simulink model "rtds"  (R2015a)
settings: Solver=ode45  StartTime=0.0  StopTime=100.0  RelTol=1e-3
undefined symbols (not defined in the file): AXI4, Lite
libraries: xbsIndex_r4 x73, s2ss x1
Description:
  | This is my first test model!
settings Model: Creator=ACS  LastModifiedBy=ACS

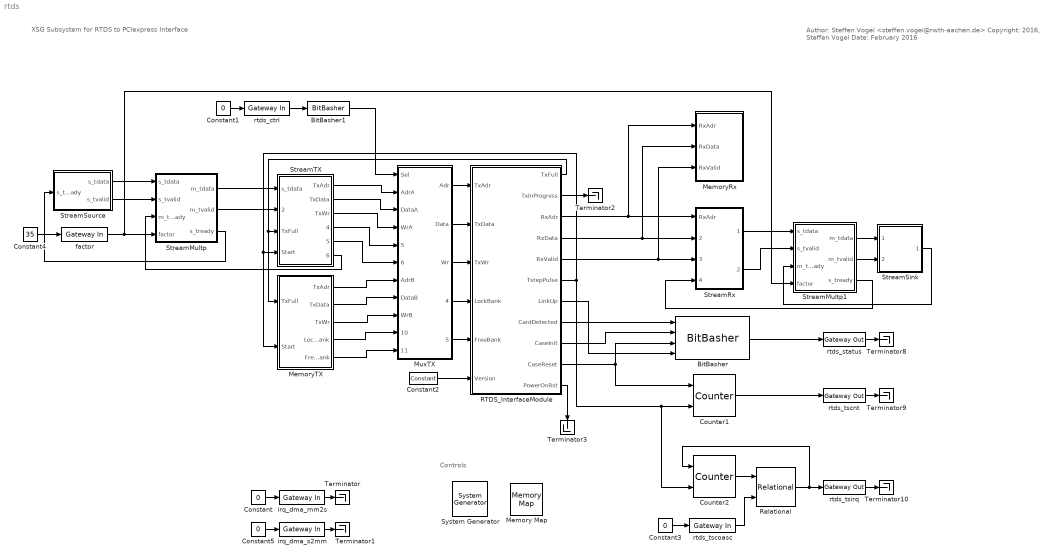
== system rtds ==
  note: XSG Subsystem for RTDS to PCIexpress Interface
  note: Author: Steffen Vogel <steffen.vogel@rwth-aachen.de>
      | Copyright: 2016, Steffen Vogel
      | Date: February 2016
  note: Controls
  " System Generator" : xbsIndex_r4/ System Generator  Tag=genX  xilinxfamily=virtex7  part=xc7vx485t  speed=-2  package=ffg1761  synthesis_tool=Vivado  clock_wrapper=Clock Enables  directory=D:/msv/02_msv-svo/s2ss/clients/sysgen/example/compiled/rtds2  proj_type=Vivado  Synth_file=Vivado Synthesis Defaults  Impl_file=Vivado Implementation Defaults  testbench=off  simulink_period=1  sysclk_period=8  dcm_input_clock_period=10  incr_netlist=off  trim_vbits=Everywhere in SubSystem  dbl_ovrd=According to Block Masks  core_generation=According to Block Masks  run_coregen=off  deprecated_control=off  eval_field=0  block_type=sysgen
  BitBasher : xbsIndex_r4/BitBasher  bitexpr=status={link_up,card_detected,case_reset,case_init}  display_expr=off  sr_1=status  arith_type1=Unsigned  bin_pt1=0  sr_2=2  arith_type2=Unsigned  bin_pt2=0  sr_3=3  arith_type3=Unsigned  bin_pt3=0  sr_4=4  arith_type4=Unsigned  bin_pt4=0  dbl_ovrd=off  block_type=bitbasher
  BitBasher1 : xbsIndex_r4/BitBasher  bitexpr=sel={ctrl[0]}  display_expr=off  sr_1=sel  arith_type1=Unsigned  bin_pt1=0  sr_2=2  arith_type2=Unsigned  bin_pt2=0  sr_3=3  arith_type3=Unsigned  bin_pt3=0  sr_4=4  arith_type4=Unsigned  bin_pt4=0  dbl_ovrd=off  block_type=bitbasher
  Constant{,1,3,5} (4 alike) : Constant  Value=0
  Constant2 : xbsIndex_r4/Constant  const=3  gui_display_data_type=Fixed-point  arith_type=Signed (2's comp)  n_bits=16  bin_pt=0  preci_type=Single  exp_width=8  frac_width=24  explicit_period=off  period=1  equ=P=C  opselect=C  inp2=PCIN>>17  opr=+  inp1=P  carry=CIN  dbl_ovrd=off  block_type=constant
  Constant4 : Constant  Value=35
  Counter1 : xbsIndex_r4/Counter  cnt_type=Free Running  cnt_to=Inf  operation=Up  start_count=0  cnt_by_val=1  arith_type=Unsigned  n_bits=32  bin_pt=0  load_pin=off  rst=on  en=on  explicit_period=on  period=1  use_behavioral_HDL=off  implementation=Fabric  dbl_ovrd=off  block_type=counter
  Counter2 : xbsIndex_r4/Counter  cnt_type=Free Running  cnt_to=Inf  operation=Up  start_count=0  cnt_by_val=1  arith_type=Unsigned  n_bits=32  bin_pt=0  load_pin=off  rst=on  en=on  explicit_period=on  period=1  use_behavioral_HDL=off  implementation=Fabric  dbl_ovrd=off  block_type=counter
  Memory Map : s2ss/Memory Map  version=1.0  author=Steffen Vogel <stvogel@eonerc.rwth-aachen.de>  desc=System Generator Model  company_url=http://www.acs.eonerc.rwth-aachen.de  vendor=acs.eonerc.rwth-aachen.de  vendor_display_name=Institute for Automation of Complex Power Systems, EONERC, RWTH Aachen University
  MemoryRx : Subsystem
  MemoryTX : Subsystem
  MuxTX : Subsystem
  RTDS_InterfaceModule : Subsystem
  Relational : xbsIndex_r4/Relational  mode=a=b  op_type=Bool  en=off  latency=1  dbl_ovrd=off  block_type=relational
  StreamMultp : Subsystem
  StreamMultp1 : Subsystem
  StreamRx : Subsystem
  StreamSink : Subsystem
  StreamSource : Subsystem
  StreamTX : Subsystem
  Terminator{,1..3,8..10} (7 alike) : Terminator
  factor : xbsIndex_r4/Gateway In  gui_display_data_type=Floating-point  arith_type=Floating-point  n_bits=32  bin_pt=0  preci_type=Single  exp_width=8  frac_width=24  rows=1  columns=1  quantization=Truncate  overflow=Wrap  period=1  UseAsADC=off  ADCChannel='1'  interface=AXI4-Lite  automatic_assignment=on  address_offset=hex2dec('00')  intf_name=''  intf_description=''  timing_constraint=None  locs_specified=off  LOCs={}  io_standard={}  inherit_from_input=off  hdl_port=on  dbl_ovrd=off  block_type=gatewayin
  irq_dma_mm2s : xbsIndex_r4/Gateway In  gui_display_data_type=Boolean  arith_type=Boolean  n_bits=32  bin_pt=0  preci_type=Single  exp_width=8  frac_width=24  rows=1  columns=1  quantization="Round  (unbiased: +/- Inf)"  overflow=Saturate  period=1  UseAsADC=off  ADCChannel='1'  interface=None  automatic_assignment=on  address_offset=hex2dec('00')  intf_name=''  intf_description=''  timing_constraint=None  locs_specified=off  LOCs={}  io_standard={}  inherit_from_input=off  hdl_port=on  dbl_ovrd=off  block_type=gatewayin
  irq_dma_s2mm : xbsIndex_r4/Gateway In  gui_display_data_type=Boolean  arith_type=Boolean  n_bits=32  bin_pt=0  preci_type=Single  exp_width=8  frac_width=24  rows=1  columns=1  quantization="Round  (unbiased: +/- Inf)"  overflow=Saturate  period=1  UseAsADC=off  ADCChannel='1'  interface=None  automatic_assignment=on  address_offset=hex2dec('00')  intf_name=''  intf_description=''  timing_constraint=None  locs_specified=off  LOCs={}  io_standard={}  inherit_from_input=off  hdl_port=on  dbl_ovrd=off  block_type=gatewayin
  rtds_ctrl : xbsIndex_r4/Gateway In  gui_display_data_type=Fixed-point  arith_type=Unsigned  n_bits=32  bin_pt=0  preci_type=Single  exp_width=8  frac_width=24  rows=1  columns=1  quantization="Round  (unbiased: +/- Inf)"  overflow=Saturate  period=1  UseAsADC=off  ADCChannel='1'  interface=AXI4-Lite  automatic_assignment=on  address_offset=hex2dec('00')  intf_name=''  intf_description=''  timing_constraint=None  locs_specified=off  LOCs={}  io_standard={}  inherit_from_input=off  hdl_port=on  dbl_ovrd=off  block_type=gatewayin
  rtds_status : xbsIndex_r4/Gateway Out  inherit_from_input=off  hdl_port=on  rows=1  columns=1  UseAsDAC=off  DACChannel='1'  interface=AXI4-Lite  automatic_assignment=on  address_offset=hex2dec('00')  intf_name=''  intf_description=''  timing_constraint=None  locs_specified=off  LOCs={}  io_standard={}  block_type=gatewayout
  rtds_tscnt : xbsIndex_r4/Gateway Out  inherit_from_input=off  hdl_port=on  rows=1  columns=1  UseAsDAC=off  DACChannel='1'  interface=AXI4-Lite  automatic_assignment=on  address_offset=hex2dec('00')  intf_name=''  intf_description=''  timing_constraint=None  locs_specified=off  LOCs={}  io_standard={}  block_type=gatewayout
  rtds_tscoasc : xbsIndex_r4/Gateway In  gui_display_data_type=Fixed-point  arith_type=Unsigned  n_bits=32  bin_pt=0  preci_type=Single  exp_width=8  frac_width=24  rows=1  columns=1  quantization=Truncate  overflow=Wrap  period=1  UseAsADC=off  ADCChannel='1'  interface=AXI4-Lite  automatic_assignment=on  address_offset=hex2dec('00')  intf_name=''  intf_description=''  timing_constraint=None  locs_specified=off  LOCs={}  io_standard={}  inherit_from_input=off  hdl_port=on  dbl_ovrd=off  block_type=gatewayin
  rtds_tsirq : xbsIndex_r4/Gateway Out  inherit_from_input=off  hdl_port=on  rows=1  columns=1  UseAsDAC=off  DACChannel='1'  interface=Interrupt  automatic_assignment=on  address_offset=hex2dec('00')  intf_name=''  intf_description=''  timing_constraint=None  locs_specified=off  LOCs={}  io_standard={}  block_type=gatewayout
  wires:
  irq_dma_mm2s/1 -> Terminator/1
  RTDS_InterfaceModule/5(RxValid) -> StreamRx/3(RxValid), MemoryRx/3(RxValid)
  BitBasher/1 -> rtds_status/1
  Counter1/1 -> rtds_tscnt/1
  Relational/1 -> Counter2/1, rtds_tsirq/1
  Counter2/1 -> Relational/1
  rtds_tscoasc/1 -> Relational/2
  RTDS_InterfaceModule/10(CaseReset) -> Counter1/1, BitBasher/3
  RTDS_InterfaceModule/4(RxData) -> MemoryRx/2(RxData), StreamRx/2(RxData)
  RTDS_InterfaceModule/8(CardDetected) -> BitBasher/1
  RTDS_InterfaceModule/9(CaseInit) -> BitBasher/2
  RTDS_InterfaceModule/7(LinkUp) -> BitBasher/4
  Constant2/1 -> RTDS_InterfaceModule/6(Version)
  RTDS_InterfaceModule/3(RxAdr) -> MemoryRx/1(RxAdr), StreamRx/1(RxAdr)
  RTDS_InterfaceModule/2(TxInProgress) -> Terminator2/1
  RTDS_InterfaceModule/11(PowerOnRst) -> Terminator3/1
  rtds_status/1 -> Terminator8/1
  rtds_tscnt/1 -> Terminator9/1
  rtds_tsirq/1 -> Terminator10/1
  rtds_ctrl/1 -> BitBasher1/1
  StreamTX/1(TxAdr) -> MuxTX/2(AdrA)
  StreamTX/2(TxData) -> MuxTX/3(DataA)
  StreamTX/3(TxWr) -> MuxTX/4(WrA)
  StreamTX/4(LockBank) -> MuxTX/5(LockBankA)
  StreamTX/5(FreeBank) -> MuxTX/6(FreeBankA)
  BitBasher1/1 -> MuxTX/1(Sel)
  MemoryTX/1(TxAdr) -> MuxTX/7(AdrB)
  MemoryTX/2(TxData) -> MuxTX/8(DataB)
  MemoryTX/3(TxWr) -> MuxTX/9(WrB)
  MemoryTX/4(LockBank) -> MuxTX/10(LockBankB)
  MemoryTX/5(FreeBank) -> MuxTX/11(FreeBankB)
  MuxTX/1(Adr) -> RTDS_InterfaceModule/1(TxAdr)
  MuxTX/2(Data) -> RTDS_InterfaceModule/2(TxData)
  MuxTX/3(Wr) -> RTDS_InterfaceModule/3(TxWr)
  MuxTX/4(LockBank) -> RTDS_InterfaceModule/4(LockBank)
  MuxTX/5(FreeBank) -> RTDS_InterfaceModule/5(FreeBank)
  RTDS_InterfaceModule/6(TstepPulse) -> Counter2/2, Counter1/2, MemoryTX/2(Start), StreamTX/4(Start)
  RTDS_InterfaceModule/1(TxFull) -> MemoryTX/1(TxFull), StreamTX/3(TxFull)
  StreamSource/1(s_tdata) -> StreamMultp/1(s_tdata)
  StreamSource/2(s_tvalid) -> StreamMultp/2(s_tvalid)
  StreamMultp/1(m_tdata) -> StreamTX/1(s_tdata)
  StreamMultp/2(m_tvalid) -> StreamTX/2(s_tvalid)
  StreamTX/6(s_tready) -> StreamMultp/3(m_tready)
  StreamMultp/3(s_tready) -> StreamSource/1(s_tready)
  StreamRx/2(m_tvalid) -> StreamMultp1/2(s_tvalid)
  StreamRx/1(m_tdata) -> StreamMultp1/1(s_tdata)
  StreamMultp1/1(m_tdata) -> StreamSink/1(s_tdata)
  StreamMultp1/2(m_tvalid) -> StreamSink/2(s_tvalid)
  StreamSink/1(s_tready) -> StreamMultp1/3(m_tready)
  factor/1 -> StreamMultp1/4(factor), StreamMultp/4(factor)
  StreamMultp1/3(s_tready) -> StreamRx/4(m_tready)
  Constant/1 -> irq_dma_mm2s/1
  Constant1/1 -> rtds_ctrl/1
  Constant3/1 -> rtds_tscoasc/1
  Constant4/1 -> factor/1
  irq_dma_s2mm/1 -> Terminator1/1
  Constant5/1 -> irq_dma_s2mm/1

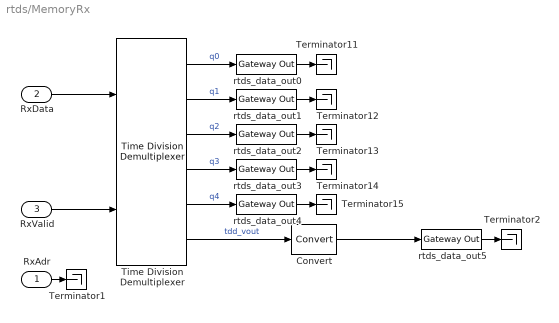
== system rtds/MemoryRx ==
  RxAdr : Inport
  RxData : Inport  Port=2
  RxValid : Inport  Port=3
  Convert : xbsIndex_r4/Convert  gui_display_data_type=Fixed-point  arith_type=Unsigned  n_bits=32  bin_pt=0  float_type=Single  exp_bits=8  fraction_bits=24  quantization=Truncate  overflow=Wrap  en=off  latency=0  pipeline=off  dbl_ovrd=off  block_type=convert
  Terminator{1..2,11..15} (7 alike) : Terminator
  Time Division Demultiplexer : xbsIndex_r4/Time Division Demultiplexer  frame_pattern=[1 1 1 1 1]  impl_style=Multiple Channel  vin=on  explicit_period=off  dbl_ovrd=off  period=1  block_type=tdd
      settings: infoedit=Samples presented at the input are selected and down-sampled according to the frame sampling pattern specified. The sampled input is presented either as a single or multiple channel at the output.
  rtds_data_out{0..5} (6 alike) : xbsIndex_r4/Gateway Out  inherit_from_input=off  hdl_port=on  rows=1  columns=1  UseAsDAC=off  DACChannel='1'  interface=AXI4-Lite  automatic_assignment=on  address_offset=hex2dec('00')  intf_name=''  intf_description=''  timing_constraint=None  locs_specified=off  LOCs={}  io_standard={}  block_type=gatewayout
  wires:
  Time Division Demultiplexer/4 -> rtds_data_out3/1  "q3"
  Time Division Demultiplexer/1 -> rtds_data_out0/1  "q0"
  rtds_data_out2/1 -> Terminator13/1
  rtds_data_out1/1 -> Terminator12/1
  Time Division Demultiplexer/2 -> rtds_data_out1/1  "q1"
  rtds_data_out3/1 -> Terminator14/1
  Time Division Demultiplexer/5 -> rtds_data_out4/1  "q4"
  Time Division Demultiplexer/3 -> rtds_data_out2/1  "q2"
  rtds_data_out4/1 -> Terminator15/1
  rtds_data_out0/1 -> Terminator11/1
  RxData/1 -> Time Division Demultiplexer/1
  RxValid/1 -> Time Division Demultiplexer/2
  RxAdr/1 -> Terminator1/1
  rtds_data_out5/1 -> Terminator2/1
  Time Division Demultiplexer/6 -> Convert/1  "tdd_vout"
  Convert/1 -> rtds_data_out5/1

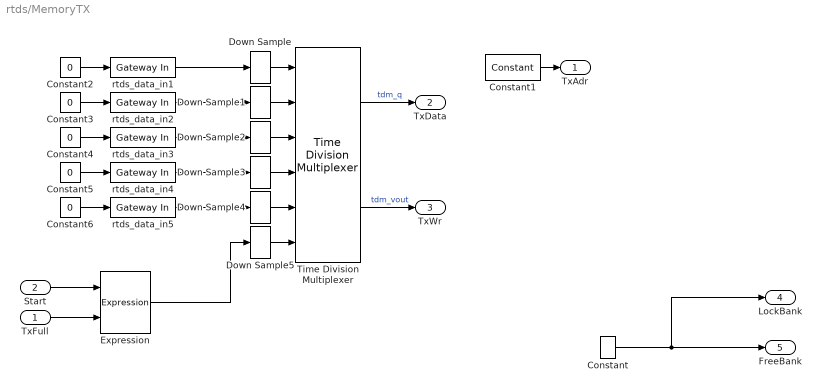
== system rtds/MemoryTX ==
  TxFull : Inport
  Start : Inport  Port=2
  Constant : xbsIndex_r4/Constant  const=0  gui_display_data_type=Boolean  arith_type=Boolean  n_bits=16  bin_pt=14  preci_type=Single  exp_width=8  frac_width=24  explicit_period=off  period=1  equ=P=C  opselect=C  inp2=PCIN>>17  opr=+  inp1=P  carry=CIN  dbl_ovrd=off  block_type=constant
  Constant1 : xbsIndex_r4/Constant  const=0  gui_display_data_type=Fixed-point  arith_type=Unsigned  n_bits=8  bin_pt=0  preci_type=Single  exp_width=8  frac_width=24  explicit_period=off  period=1  equ=P=C  opselect=C  inp2=PCIN>>17  opr=+  inp1=P  carry=CIN  dbl_ovrd=off  block_type=constant
  Constant{2..6} (5 alike) : Constant  Value=0
  Down Sample{,1..5} (6 alike) : xbsIndex_r4/Down Sample  sample_ratio=5  sample_phase="Last Value of Frame  (most efficient)"  en=off  rst=off  latency=1  dbl_ovrd=off  block_type=dsamp
  Expression : xbsIndex_r4/Expression  expression=a & ~b  align_bp=on  en=off  latency=0  precision=Full  arith_type=Unsigned  n_bits=16  bin_pt=0  dbl_ovrd=off  block_type=expr
  Time Division Multiplexer : xbsIndex_r4/Time Division Multiplexer  inputs=5  vin=on  Optimization=Resource  explicit_period=off  period=1  dbl_ovrd=off  block_type=tdm
      settings: infoedit="Multiple inputs are sampled and  presented serially at the output."
  rtds_data_in1 : xbsIndex_r4/Gateway In  gui_display_data_type=Fixed-point  arith_type=Unsigned  n_bits=32  bin_pt=0  preci_type=Single  exp_width=8  frac_width=24  rows=1  columns=1  quantization="Round  (unbiased: +/- Inf)"  overflow=Saturate  period=1  UseAsADC=off  ADCChannel='1'  interface=AXI4-Lite  automatic_assignment=on  address_offset=hex2dec('00')  intf_name=''  intf_description=''  timing_constraint=None  locs_specified=off  LOCs={}  io_standard={}  inherit_from_input=off  hdl_port=on  dbl_ovrd=off  block_type=gatewayin
  rtds_data_in2 : xbsIndex_r4/Gateway In  gui_display_data_type=Fixed-point  arith_type=Unsigned  n_bits=32  bin_pt=0  preci_type=Single  exp_width=8  frac_width=24  rows=1  columns=1  quantization="Round  (unbiased: +/- Inf)"  overflow=Saturate  period=1  UseAsADC=off  ADCChannel='1'  interface=AXI4-Lite  automatic_assignment=on  address_offset=hex2dec('00')  intf_name=''  intf_description=''  timing_constraint=None  locs_specified=off  LOCs={}  io_standard={}  inherit_from_input=off  hdl_port=on  dbl_ovrd=off  block_type=gatewayin
  rtds_data_in3 : xbsIndex_r4/Gateway In  gui_display_data_type=Fixed-point  arith_type=Unsigned  n_bits=32  bin_pt=0  preci_type=Single  exp_width=8  frac_width=24  rows=1  columns=1  quantization="Round  (unbiased: +/- Inf)"  overflow=Saturate  period=1  UseAsADC=off  ADCChannel='1'  interface=AXI4-Lite  automatic_assignment=on  address_offset=hex2dec('00')  intf_name=''  intf_description=''  timing_constraint=None  locs_specified=off  LOCs={}  io_standard={}  inherit_from_input=off  hdl_port=on  dbl_ovrd=off  block_type=gatewayin
  rtds_data_in4 : xbsIndex_r4/Gateway In  gui_display_data_type=Fixed-point  arith_type="Signed  (2's comp)"  n_bits=32  bin_pt=6  preci_type=Single  exp_width=8  frac_width=24  rows=1  columns=1  quantization="Round  (unbiased: +/- Inf)"  overflow=Saturate  period=1  UseAsADC=off  ADCChannel='1'  interface=AXI4-Lite  automatic_assignment=on  address_offset=hex2dec('00')  intf_name=''  intf_description=''  timing_constraint=None  locs_specified=off  LOCs={}  io_standard={}  inherit_from_input=off  hdl_port=on  dbl_ovrd=off  block_type=gatewayin
  rtds_data_in5 : xbsIndex_r4/Gateway In  gui_display_data_type=Boolean  arith_type=Boolean  n_bits=32  bin_pt=0  preci_type=Single  exp_width=8  frac_width=24  rows=1  columns=1  quantization="Round  (unbiased: +/- Inf)"  overflow=Saturate  period=1  UseAsADC=off  ADCChannel='1'  interface=AXI4-Lite  automatic_assignment=on  address_offset=hex2dec('00')  intf_name=''  intf_description=''  timing_constraint=None  locs_specified=off  LOCs={}  io_standard={}  inherit_from_input=off  hdl_port=on  dbl_ovrd=off  block_type=gatewayin
  TxAdr : Outport
  TxData : Outport  Port=2
  TxWr : Outport  Port=3
  LockBank : Outport  Port=4
  FreeBank : Outport  Port=5
  wires:
  rtds_data_in1/1 -> Down Sample/1
  rtds_data_in4/1 -> Down Sample3/1
  Time Division Multiplexer/2 -> TxWr/1  "tdm_vout"
  Time Division Multiplexer/1 -> TxData/1  "tdm_q"
  rtds_data_in5/1 -> Down Sample4/1
  rtds_data_in2/1 -> Down Sample1/1
  rtds_data_in3/1 -> Down Sample2/1
  Constant/1 -> LockBank/1, FreeBank/1
  Down Sample/1 -> Time Division Multiplexer/1
  Down Sample1/1 -> Time Division Multiplexer/2
  Down Sample2/1 -> Time Division Multiplexer/3
  Down Sample3/1 -> Time Division Multiplexer/4
  Down Sample4/1 -> Time Division Multiplexer/5
  Down Sample5/1 -> Time Division Multiplexer/6
  TxFull/1 -> Expression/2
  Start/1 -> Expression/1
  Expression/1 -> Down Sample5/1
  Constant1/1 -> TxAdr/1
  Constant6/1 -> rtds_data_in5/1
  Constant5/1 -> rtds_data_in4/1
  Constant4/1 -> rtds_data_in3/1
  Constant3/1 -> rtds_data_in2/1
  Constant2/1 -> rtds_data_in1/1

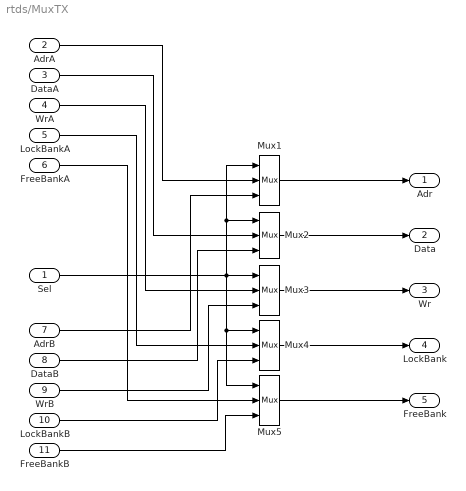
== system rtds/MuxTX ==
  Sel : Inport
  AdrA : Inport  Port=2
  DataA : Inport  Port=3
  WrA : Inport  Port=4
  LockBankA : Inport  Port=5
  FreeBankA : Inport  Port=6
  AdrB : Inport  Port=7
  DataB : Inport  Port=8
  WrB : Inport  Port=9
  LockBankB : Inport  Port=10
  FreeBankB : Inport  Port=11
  Mux{1..5} (5 alike) : xbsIndex_r4/Mux  inputs=2  en=off  latency=0  precision=Full  arith_type=Unsigned  n_bits=16  bin_pt=14  quantization=Truncate  overflow=Wrap  dbl_ovrd=off  block_type=mux
  Adr : Outport
  Data : Outport  Port=2
  Wr : Outport  Port=3
  LockBank : Outport  Port=4
  FreeBank : Outport  Port=5
  wires:
  AdrB/1 -> Mux1/3
  WrA/1 -> Mux3/2
  DataB/1 -> Mux2/3
  WrB/1 -> Mux3/3
  AdrA/1 -> Mux1/2
  DataA/1 -> Mux2/2
  Mux5/1 -> FreeBank/1
  Mux4/1 -> LockBank/1
  Mux3/1 -> Wr/1
  Mux1/1 -> Adr/1
  Sel/1 -> Mux3/1, Mux5/1, Mux4/1, Mux1/1, Mux2/1
  Mux2/1 -> Data/1
  LockBankA/1 -> Mux4/2
  FreeBankB/1 -> Mux5/3
  FreeBankA/1 -> Mux5/2
  LockBankB/1 -> Mux4/3

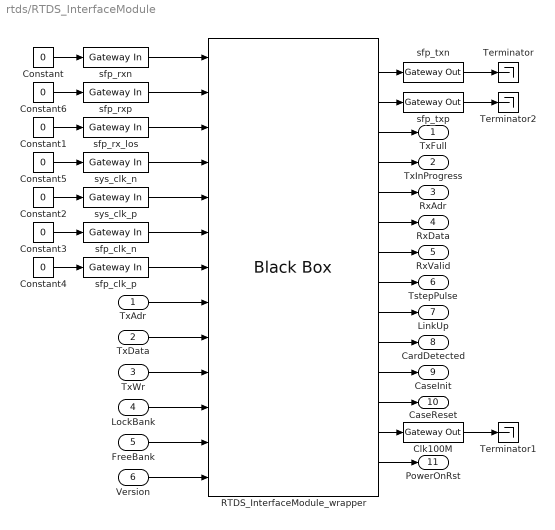
== system rtds/RTDS_InterfaceModule ==
  TxAdr : Inport
  TxData : Inport  Port=2
  TxWr : Inport  Port=3
  LockBank : Inport  Port=4
  FreeBank : Inport  Port=5
  Version : Inport  Port=6
  Clk100M : xbsIndex_r4/Gateway Out  inherit_from_input=off  hdl_port=on  rows=1  columns=1  UseAsDAC=off  DACChannel='1'  interface=None  automatic_assignment=on  address_offset=hex2dec('00')  intf_name=''  intf_description=''  timing_constraint=None  locs_specified=off  LOCs={}  io_standard={}  block_type=gatewayout
  Constant{,1..6} (7 alike) : Constant  Value=0
  RTDS_InterfaceModule_wrapper : xbsIndex_r4/Black Box  init_code=RTDS_InterfaceModule_wrapper_config  sim_method=ISE Simulator  verbose=off  block_type=blackbox2
  Terminator : Terminator
  Terminator1 : Terminator
  Terminator2 : Terminator
  sfp_clk_n : xbsIndex_r4/Gateway In  gui_display_data_type=Boolean  arith_type=Boolean  n_bits=2  bin_pt=0  preci_type=Single  exp_width=8  frac_width=24  rows=1  columns=1  quantization=Truncate  overflow=Wrap  period=1  UseAsADC=off  ADCChannel='1'  interface=None  automatic_assignment=on  address_offset=hex2dec('00')  intf_name=''  intf_description=''  timing_constraint=None  locs_specified=off  LOCs={}  io_standard={}  inherit_from_input=off  hdl_port=on  dbl_ovrd=off  block_type=gatewayin
  sfp_clk_p : xbsIndex_r4/Gateway In  gui_display_data_type=Boolean  arith_type=Boolean  n_bits=2  bin_pt=0  preci_type=Single  exp_width=8  frac_width=24  rows=1  columns=1  quantization=Truncate  overflow=Wrap  period=1  UseAsADC=off  ADCChannel='1'  interface=None  automatic_assignment=on  address_offset=hex2dec('00')  intf_name=''  intf_description=''  timing_constraint=None  locs_specified=off  LOCs={}  io_standard={}  inherit_from_input=off  hdl_port=on  dbl_ovrd=off  block_type=gatewayin
  sfp_rx_los : xbsIndex_r4/Gateway In  gui_display_data_type=Boolean  arith_type=Boolean  n_bits=16  bin_pt=14  preci_type=Single  exp_width=8  frac_width=24  rows=1  columns=1  quantization="Round  (unbiased: +/- Inf)"  overflow=Saturate  period=1  UseAsADC=off  ADCChannel='1'  interface=None  automatic_assignment=on  address_offset=hex2dec('00')  intf_name=''  intf_description=''  timing_constraint=None  locs_specified=off  LOCs={}  io_standard={}  inherit_from_input=off  hdl_port=on  dbl_ovrd=off  block_type=gatewayin
  sfp_rxn : xbsIndex_r4/Gateway In  gui_display_data_type=Boolean  arith_type=Boolean  n_bits=2  bin_pt=0  preci_type=Single  exp_width=8  frac_width=24  rows=1  columns=1  quantization=Truncate  overflow=Wrap  period=1  UseAsADC=off  ADCChannel='1'  interface=None  automatic_assignment=on  address_offset=hex2dec('00')  intf_name=''  intf_description=''  timing_constraint=None  locs_specified=off  LOCs={}  io_standard={}  inherit_from_input=off  hdl_port=on  dbl_ovrd=off  block_type=gatewayin
  sfp_rxp : xbsIndex_r4/Gateway In  gui_display_data_type=Boolean  arith_type=Boolean  n_bits=2  bin_pt=0  preci_type=Single  exp_width=8  frac_width=24  rows=1  columns=1  quantization=Truncate  overflow=Wrap  period=1  UseAsADC=off  ADCChannel='1'  interface=None  automatic_assignment=on  address_offset=hex2dec('00')  intf_name=''  intf_description=''  timing_constraint=None  locs_specified=off  LOCs={}  io_standard={}  inherit_from_input=off  hdl_port=on  dbl_ovrd=off  block_type=gatewayin
  sfp_txn : xbsIndex_r4/Gateway Out  inherit_from_input=off  hdl_port=on  rows=1  columns=1  UseAsDAC=off  DACChannel='1'  interface=None  automatic_assignment=on  address_offset=hex2dec('00')  intf_name=''  intf_description=''  timing_constraint=None  locs_specified=off  LOCs={}  io_standard={}  block_type=gatewayout
  sfp_txp : xbsIndex_r4/Gateway Out  inherit_from_input=off  hdl_port=on  rows=1  columns=1  UseAsDAC=off  DACChannel='1'  interface=None  automatic_assignment=on  address_offset=hex2dec('00')  intf_name=''  intf_description=''  timing_constraint=None  locs_specified=off  LOCs={}  io_standard={}  block_type=gatewayout
  sys_clk_n : xbsIndex_r4/Gateway In  gui_display_data_type=Boolean  arith_type=Boolean  n_bits=2  bin_pt=0  preci_type=Single  exp_width=8  frac_width=24  rows=1  columns=1  quantization=Truncate  overflow=Wrap  period=1  UseAsADC=off  ADCChannel='1'  interface=None  automatic_assignment=on  address_offset=hex2dec('00')  intf_name=''  intf_description=''  timing_constraint=None  locs_specified=off  LOCs={}  io_standard={}  inherit_from_input=off  hdl_port=on  dbl_ovrd=off  block_type=gatewayin
  sys_clk_p : xbsIndex_r4/Gateway In  gui_display_data_type=Boolean  arith_type=Boolean  n_bits=2  bin_pt=0  preci_type=Single  exp_width=8  frac_width=24  rows=1  columns=1  quantization=Truncate  overflow=Wrap  period=1  UseAsADC=off  ADCChannel='1'  interface=None  automatic_assignment=on  address_offset=hex2dec('00')  intf_name=''  intf_description=''  timing_constraint=None  locs_specified=off  LOCs={}  io_standard={}  inherit_from_input=off  hdl_port=on  dbl_ovrd=off  block_type=gatewayin
  TxFull : Outport
  TxInProgress : Outport  Port=2
  RxAdr : Outport  Port=3
  RxData : Outport  Port=4
  RxValid : Outport  Port=5
  TstepPulse : Outport  Port=6
  LinkUp : Outport  Port=7
  CardDetected : Outport  Port=8
  CaseInit : Outport  Port=9
  CaseReset : Outport  Port=10
  PowerOnRst : Outport  Port=11
  wires:
  sfp_rxn/1 -> RTDS_InterfaceModule_wrapper/1
  RTDS_InterfaceModule_wrapper/1 -> sfp_txn/1
  sfp_txn/1 -> Terminator/1
  Constant/1 -> sfp_rxn/1
  Constant1/1 -> sfp_rx_los/1
  Constant2/1 -> sys_clk_p/1
  Constant3/1 -> sfp_clk_n/1
  Version/1 -> RTDS_InterfaceModule_wrapper/13
  FreeBank/1 -> RTDS_InterfaceModule_wrapper/12
  LockBank/1 -> RTDS_InterfaceModule_wrapper/11
  TxWr/1 -> RTDS_InterfaceModule_wrapper/10
  TxData/1 -> RTDS_InterfaceModule_wrapper/9
  TxAdr/1 -> RTDS_InterfaceModule_wrapper/8
  sfp_clk_n/1 -> RTDS_InterfaceModule_wrapper/6
  sfp_clk_p/1 -> RTDS_InterfaceModule_wrapper/7
  Constant4/1 -> sfp_clk_p/1
  sys_clk_p/1 -> RTDS_InterfaceModule_wrapper/5
  sys_clk_n/1 -> RTDS_InterfaceModule_wrapper/4
  sfp_rx_los/1 -> RTDS_InterfaceModule_wrapper/3
  sfp_rxp/1 -> RTDS_InterfaceModule_wrapper/2
  RTDS_InterfaceModule_wrapper/14 -> PowerOnRst/1
  RTDS_InterfaceModule_wrapper/12 -> CaseReset/1
  RTDS_InterfaceModule_wrapper/11 -> CaseInit/1
  RTDS_InterfaceModule_wrapper/10 -> CardDetected/1
  RTDS_InterfaceModule_wrapper/9 -> LinkUp/1
  RTDS_InterfaceModule_wrapper/8 -> TstepPulse/1
  RTDS_InterfaceModule_wrapper/7 -> RxValid/1
  RTDS_InterfaceModule_wrapper/6 -> RxData/1
  RTDS_InterfaceModule_wrapper/5 -> RxAdr/1
  RTDS_InterfaceModule_wrapper/4 -> TxInProgress/1
  RTDS_InterfaceModule_wrapper/3 -> TxFull/1
  RTDS_InterfaceModule_wrapper/2 -> sfp_txp/1
  sfp_txp/1 -> Terminator2/1
  Constant6/1 -> sfp_rxp/1
  Constant5/1 -> sys_clk_n/1
  RTDS_InterfaceModule_wrapper/13 -> Clk100M/1
  Clk100M/1 -> Terminator1/1

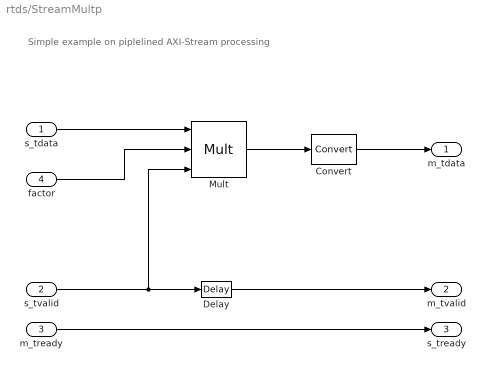
== system rtds/StreamMultp ==
  note: Simple example on piplelined AXI-Stream processing
  s_tdata : Inport
  s_tvalid : Inport  Port=2
  m_tready : Inport  Port=3
  factor : Inport  Port=4
  Convert : xbsIndex_r4/Convert  gui_display_data_type=Fixed-point  arith_type=Unsigned  n_bits=32  bin_pt=0  float_type=Single  exp_bits=8  fraction_bits=24  quantization=Truncate  overflow=Wrap  en=off  latency=0  pipeline=off  dbl_ovrd=off  block_type=convert
  Delay : xbsIndex_r4/Delay  rst=off  infoeditControl=Selection of Reset will increase slice count due to use of real FFs and instead of SRLs  en=off  latency=3  reg_retiming=off  dbl_ovrd=off  block_type=delay
  Mult : xbsIndex_r4/Mult  precision=Full  arith_type="Signed  (2's comp)"  n_bits=16  bin_pt=14  quantization=Truncate  overflow=Wrap  en=on  latency=3  use_behavioral_HDL=off  opt=Speed  use_embedded=on  optimum_pipeline=off  pipeline=on  dbl_ovrd=off  use_rpm=on  placement_style=Triangular  block_type=mult
  m_tdata : Outport
  m_tvalid : Outport  Port=2
  s_tready : Outport  Port=3
  wires:
  factor/1 -> Mult/2
  Mult/1 -> Convert/1
  s_tdata/1 -> Mult/1
  s_tvalid/1 -> Delay/1, Mult/3
  Delay/1 -> m_tvalid/1
  m_tready/1 -> s_tready/1
  Convert/1 -> m_tdata/1

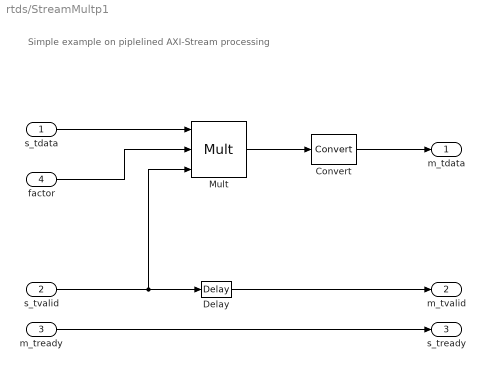
== system rtds/StreamMultp1 ==
  note: Simple example on piplelined AXI-Stream processing
  s_tdata : Inport
  s_tvalid : Inport  Port=2
  m_tready : Inport  Port=3
  factor : Inport  Port=4
  Convert : xbsIndex_r4/Convert  gui_display_data_type=Fixed-point  arith_type=Unsigned  n_bits=32  bin_pt=0  float_type=Single  exp_bits=8  fraction_bits=24  quantization=Truncate  overflow=Wrap  en=off  latency=0  pipeline=off  dbl_ovrd=off  block_type=convert
  Delay : xbsIndex_r4/Delay  rst=off  infoeditControl=Selection of Reset will increase slice count due to use of real FFs and instead of SRLs  en=off  latency=3  reg_retiming=off  dbl_ovrd=off  block_type=delay
  Mult : xbsIndex_r4/Mult  precision=Full  arith_type="Signed  (2's comp)"  n_bits=16  bin_pt=14  quantization=Truncate  overflow=Wrap  en=on  latency=3  use_behavioral_HDL=off  opt=Speed  use_embedded=on  optimum_pipeline=off  pipeline=on  dbl_ovrd=off  use_rpm=on  placement_style=Triangular  block_type=mult
  m_tdata : Outport
  m_tvalid : Outport  Port=2
  s_tready : Outport  Port=3
  wires:
  factor/1 -> Mult/2
  Mult/1 -> Convert/1
  s_tdata/1 -> Mult/1
  s_tvalid/1 -> Delay/1, Mult/3
  Delay/1 -> m_tvalid/1
  m_tready/1 -> s_tready/1
  Convert/1 -> m_tdata/1

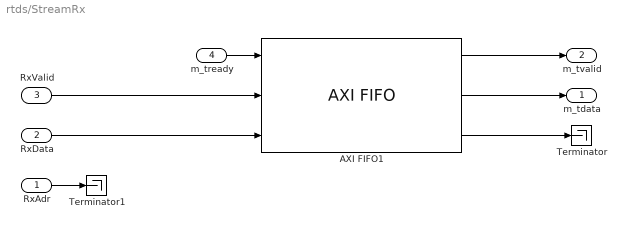
== system rtds/StreamRx ==
  RxAdr : Inport
  RxData : Inport  Port=2
  RxValid : Inport  Port=3
  m_tready : Inport  Port=4
  AXI FIFO1 : xbsIndex_r4/AXI FIFO  input_depth_axis=512  actual_fifo_depth_label=514  enable_tdata=on  enable_tdest=off  enable_tstrb=off  enable_tready=on  enable_tid=off  enable_tuser=off  enable_tkeep=off  enable_tlast=off  has_aresetn=off  enable_data_counts_axis=off  fifo_implementation_type_axis=Common Clock Block RAM  trim_axipin_name=on  programmable_full_type_axis=Full  full_threshold_assert_value_axis=0  programmable_empty_type_axis=Empty  empty_threshold_assert_value_axis=1022  underflow_flag_axi=0  underflow_sense_axi=Active High  overflow_flag_axi=0  overflow_sense_axi=Active High  block_type=axi_fifo
  Terminator : Terminator
  Terminator1 : Terminator
  m_tdata : Outport
  m_tvalid : Outport  Port=2
  wires:
  RxValid/1 -> AXI FIFO1/2
  RxData/1 -> AXI FIFO1/3
  AXI FIFO1/1 -> m_tvalid/1
  m_tready/1 -> AXI FIFO1/1
  AXI FIFO1/2 -> m_tdata/1
  AXI FIFO1/3 -> Terminator/1
  RxAdr/1 -> Terminator1/1

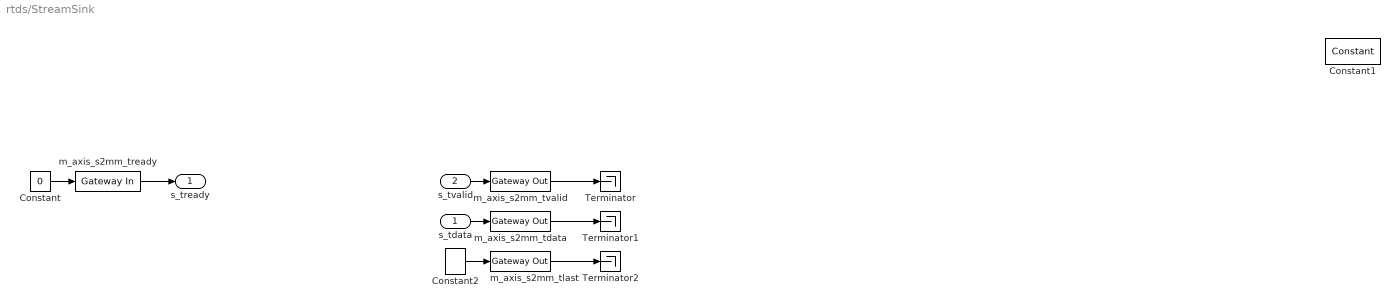
== system rtds/StreamSink ==
  s_tdata : Inport
  s_tvalid : Inport  Port=2
  Constant : Constant  Value=0
  Constant1 : xbsIndex_r4/Constant  const=1.0  gui_display_data_type=Fixed-point  arith_type=Signed (2's comp)  n_bits=16  bin_pt=14  preci_type=Single  exp_width=8  frac_width=24  explicit_period=off  period=1  equ=P=C  opselect=C  inp2=PCIN>>17  opr=+  inp1=P  carry=CIN  dbl_ovrd=off  block_type=constant
  Constant2 : xbsIndex_r4/Constant  const=0  gui_display_data_type=Boolean  arith_type=Boolean  n_bits=16  bin_pt=14  preci_type=Single  exp_width=8  frac_width=24  explicit_period=off  period=1  equ=P=C  opselect=C  inp2=PCIN>>17  opr=+  inp1=P  carry=CIN  dbl_ovrd=off  block_type=constant
  Terminator : Terminator
  Terminator1 : Terminator
  Terminator2 : Terminator
  m_axis_s2mm_tdata : xbsIndex_r4/Gateway Out  inherit_from_input=off  hdl_port=on  rows=1  columns=1  UseAsDAC=off  DACChannel='1'  interface=None  automatic_assignment=on  address_offset=hex2dec('00')  intf_name=''  intf_description=''  timing_constraint=None  locs_specified=off  LOCs={}  io_standard={}  block_type=gatewayout
  m_axis_s2mm_tlast : xbsIndex_r4/Gateway Out  inherit_from_input=off  hdl_port=on  rows=1  columns=1  UseAsDAC=off  DACChannel='1'  interface=None  automatic_assignment=on  address_offset=hex2dec('00')  intf_name=''  intf_description=''  timing_constraint=None  locs_specified=off  LOCs={}  io_standard={}  block_type=gatewayout
  m_axis_s2mm_tready : xbsIndex_r4/Gateway In  gui_display_data_type=Boolean  arith_type=Boolean  n_bits=16  bin_pt=14  preci_type=Single  exp_width=8  frac_width=24  rows=1  columns=1  quantization="Round  (unbiased: +/- Inf)"  overflow=Saturate  period=1  UseAsADC=off  ADCChannel='1'  interface=None  automatic_assignment=on  address_offset=hex2dec('00')  intf_name=''  intf_description=''  timing_constraint=None  locs_specified=off  LOCs={}  io_standard={}  inherit_from_input=off  hdl_port=on  dbl_ovrd=off  block_type=gatewayin
  m_axis_s2mm_tvalid : xbsIndex_r4/Gateway Out  inherit_from_input=off  hdl_port=on  rows=1  columns=1  UseAsDAC=off  DACChannel='1'  interface=None  automatic_assignment=on  address_offset=hex2dec('00')  intf_name=''  intf_description=''  timing_constraint=None  locs_specified=off  LOCs={}  io_standard={}  block_type=gatewayout
  s_tready : Outport
  wires:
  s_tdata/1 -> m_axis_s2mm_tdata/1
  m_axis_s2mm_tready/1 -> s_tready/1
  s_tvalid/1 -> m_axis_s2mm_tvalid/1
  m_axis_s2mm_tvalid/1 -> Terminator/1
  m_axis_s2mm_tdata/1 -> Terminator1/1
  Constant/1 -> m_axis_s2mm_tready/1
  m_axis_s2mm_tlast/1 -> Terminator2/1
  Constant2/1 -> m_axis_s2mm_tlast/1

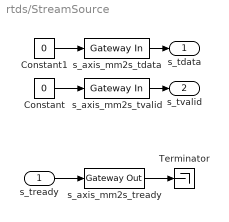
== system rtds/StreamSource ==
  s_tready : Inport
  Constant : Constant  Value=0
  Constant1 : Constant  Value=0
  Terminator : Terminator
  s_axis_mm2s_tdata : xbsIndex_r4/Gateway In  gui_display_data_type=Fixed-point  arith_type=Unsigned  n_bits=32  bin_pt=0  preci_type=Single  exp_width=8  frac_width=24  rows=1  columns=1  quantization="Round  (unbiased: +/- Inf)"  overflow=Saturate  period=1  UseAsADC=off  ADCChannel='1'  interface=None  automatic_assignment=on  address_offset=hex2dec('00')  intf_name=''  intf_description=''  timing_constraint=None  locs_specified=off  LOCs={}  io_standard={}  inherit_from_input=off  hdl_port=on  dbl_ovrd=off  block_type=gatewayin
  s_axis_mm2s_tready : xbsIndex_r4/Gateway Out  inherit_from_input=off  hdl_port=on  rows=1  columns=1  UseAsDAC=off  DACChannel='1'  interface=None  automatic_assignment=on  address_offset=hex2dec('00')  intf_name=''  intf_description=''  timing_constraint=None  locs_specified=off  LOCs={}  io_standard={}  block_type=gatewayout
  s_axis_mm2s_tvalid : xbsIndex_r4/Gateway In  gui_display_data_type=Boolean  arith_type=Boolean  n_bits=16  bin_pt=14  preci_type=Single  exp_width=8  frac_width=24  rows=1  columns=1  quantization="Round  (unbiased: +/- Inf)"  overflow=Saturate  period=1  UseAsADC=off  ADCChannel='1'  interface=None  automatic_assignment=on  address_offset=hex2dec('00')  intf_name=''  intf_description=''  timing_constraint=None  locs_specified=off  LOCs={}  io_standard={}  inherit_from_input=off  hdl_port=on  dbl_ovrd=off  block_type=gatewayin
  s_tdata : Outport
  s_tvalid : Outport  Port=2
  wires:
  s_axis_mm2s_tdata/1 -> s_tdata/1
  s_axis_mm2s_tvalid/1 -> s_tvalid/1
  s_tready/1 -> s_axis_mm2s_tready/1
  s_axis_mm2s_tready/1 -> Terminator/1
  Constant/1 -> s_axis_mm2s_tvalid/1
  Constant1/1 -> s_axis_mm2s_tdata/1

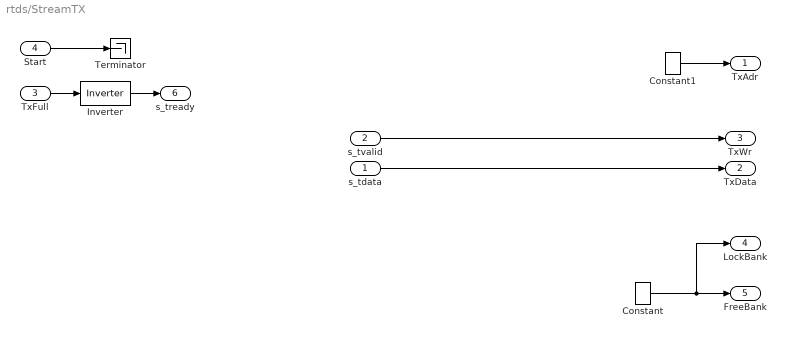
== system rtds/StreamTX ==
  s_tdata : Inport
  s_tvalid : Inport  Port=2
  TxFull : Inport  Port=3
  Start : Inport  Port=4
  Constant : xbsIndex_r4/Constant  const=0  gui_display_data_type=Boolean  arith_type=Boolean  n_bits=16  bin_pt=14  preci_type=Single  exp_width=8  frac_width=24  explicit_period=off  period=1  equ=P=C  opselect=C  inp2=PCIN>>17  opr=+  inp1=P  carry=CIN  dbl_ovrd=off  block_type=constant
  Constant1 : xbsIndex_r4/Constant  const=0  gui_display_data_type=Fixed-point  arith_type=Unsigned  n_bits=8  bin_pt=0  preci_type=Single  exp_width=8  frac_width=24  explicit_period=off  period=1  equ=P=C  opselect=C  inp2=PCIN>>17  opr=+  inp1=P  carry=CIN  dbl_ovrd=off  block_type=constant
  Inverter : xbsIndex_r4/Inverter  en=off  latency=0  dbl_ovrd=off  block_type=inv
  Terminator : Terminator
  TxAdr : Outport
  TxData : Outport  Port=2
  TxWr : Outport  Port=3
  LockBank : Outport  Port=4
  FreeBank : Outport  Port=5
  s_tready : Outport  Port=6
  wires:
  Constant/1 -> LockBank/1, FreeBank/1
  Constant1/1 -> TxAdr/1
  s_tvalid/1 -> TxWr/1
  s_tdata/1 -> TxData/1
  TxFull/1 -> Inverter/1
  Inverter/1 -> s_tready/1
  Start/1 -> Terminator/1
